simulink library "genset"  (R2014b)
settings: Solver=ode3  StartTime=0.0  StopTime=10.0  RelTol=1e-3
undefined symbols (not defined in the file): AFlowcontrol, AFn, generators, genset, i, Kappa1, ma0, magnitude, nr, pin0, swbId
libraries: goto x6, genset x3, simulink x2, switchboard x1
(part 2 of 2)

== system genset/GensetMV/Primover and generator/MVEM_TC/exhaustReceiver ==
  dm : Inport
  dE : Inport  Port=2
  dmb : Inport  Port=3
  dV : Inport  Port=4
  Bus Creator : BusCreator
  S-Function : S-Function  FunctionName=ThdynCVNV  Parameters=fs,m0,E0,mb0,V0  SFunctionModules=GetThdynCombGasZach.c GetPTF.c  EnableBusSupport=off
  pTFV : Outport
  wires:
  dE/1 -> S-Function/2
  dm/1 -> S-Function/1
  dmb/1 -> S-Function/3
  dV/1 -> S-Function/4
  S-Function/2 -> Bus Creator/2  "T"
  S-Function/1 -> Bus Creator/1  "p"
  S-Function/3 -> Bus Creator/3  "F"
  S-Function/4 -> Bus Creator/4  "V"
  Bus Creator/1 -> pTFV/1

== system genset/GensetMV/Primover and generator/MVEM_TC/pipe ==
  dm : Inport
  dE : Inport  Port=2
  dmb : Inport  Port=3
  dV : Inport  Port=4
  Bus Creator : BusCreator
  S-Function : S-Function  FunctionName=ThdynCVNV  Parameters=fs,m0,E0,mb0,V0  SFunctionModules=GetThdynCombGasZach.c GetPTF.c  EnableBusSupport=off
  pTFV : Outport
  wires:
  dE/1 -> S-Function/2
  dm/1 -> S-Function/1
  dmb/1 -> S-Function/3
  dV/1 -> S-Function/4
  S-Function/2 -> Bus Creator/2  "T"
  S-Function/1 -> Bus Creator/1  "p"
  S-Function/3 -> Bus Creator/3  "F"
  S-Function/4 -> Bus Creator/4  "V"
  Bus Creator/1 -> pTFV/1

== system genset/GensetMV/Primover and generator/Smoke Limiter MV/LP_T0_01 ==
  In1 : Inport
  Gain3 : Gain  Gain=100
  Integrator : Integrator  InitialCondition=T0AR
  Sum : Sum  Inputs=|+-
  Out1 : Outport
  wires:
  Integrator/1 -> Sum/2, Out1/1
  In1/1 -> Sum/1
  Sum/1 -> Gain3/1
  Gain3/1 -> Integrator/1

== system genset/GensetMV/Primover and generator/Smoke Limiter MV/LP_T0_1 ==
  In1 : Inport
  Gain3 : Gain  Gain=100
  Integrator : Integrator  InitialCondition=p0AR
  Sum : Sum  Inputs=|+-
  Out1 : Outport
  wires:
  Integrator/1 -> Sum/2, Out1/1
  In1/1 -> Sum/1
  Sum/1 -> Gain3/1
  Gain3/1 -> Integrator/1

== system genset/GensetMV/Primover and generator/Smoke Limiter MV/LP_T0_2 ==
  In1 : Inport
  Gain3 : Gain  Gain=100
  Integrator : Integrator  InitialCondition=p0AR/1e5*(p0AR/1e5*vol_eff_coeff(1) + vol_eff_coeff(2))+vol_eff_coeff(3)
  Sum : Sum  Inputs=|+-
  Out1 : Outport
  wires:
  Integrator/1 -> Sum/2, Out1/1
  In1/1 -> Sum/1
  Sum/1 -> Gain3/1
  Gain3/1 -> Integrator/1

== matlab function genset/GensetMV/Power calculation ==
  data: Z input; connected input; p output; E input; V input; q output; Vt output
function [p,q,Vt] = power(Z,connected,E,V)
%#codegen
if (connected)
Vt = V;
V = V/sqrt(3);
s = 3*V.*conj((E-V)./Z);
p = real(s);
q = imag(s);

else
p = 0;
q = 0;
Vt =E*sqrt(3);
end

== matlab function genset/GensetMV/Primover and generator/Electrical system ==
  data: umax input; p input size=1; q input; v input; genset_data input; te output; w input; pmax output size=1
function [te,pmax] = fcn(umax,p,q,v,genset_data,w)
r     = genset_data(1);
D     = genset_data(2);
p_max = genset_data(3);

te = (p+r*(p^2+q^2)/v^2)/w;
pmax = min((v/(1+r))*(-D*w^2+umax*w-r*q^2/v),p_max);

== matlab function genset/GensetMV/Primover and generator/Subsystem1/MATLAB Function ==
  data: u input; y output
function y = fcn(u)
%#codegen

y = anglemap(u);

== matlab function genset/GensetDC/MATLAB Function1 ==
  data: u input
function stopper(u)
%#codegen
if ( u < -1)
    error('Bus voltage calculations have been invalid for 1 second, stopping stimulation');
end

== matlab function genset/Genset/Power calculation ==
  data: Z input; connected input; p output; E input; V input; q output; Vt output
function [p,q,Vt] = power(Z,connected,E,V)
%#codegen
if (connected)
Vt = V;
V = V/sqrt(3);
s = 3*V.*conj((E-V)./Z);
p = real(s);
q = imag(s);

else
p = 0;
q = 0;
Vt =E*sqrt(3);
end

== matlab function genset/Genset/Primover and generator/Electrical system ==
  data: umax input; p input size=1; q input; v input; genset_data input; te output; w input; pmax output size=1
function [te,pmax] = fcn(umax,p,q,v,genset_data,w)
r     = genset_data(1);
D     = genset_data(2);
p_max = genset_data(3);

te = (p+r*(p^2+q^2)/v^2)/w;
pmax = min((v/(1+r))*(-D*w^2+umax*w-r*q^2/v),p_max);

== matlab function genset/Genset/Primover and generator/Subsystem1/MATLAB Function ==
  data: u input; y output
function y = fcn(u)
%#codegen

y = anglemap(u);

== matlab function genset/Genset/Primover and generator/turbo/MATLAB Function ==
  data: umax output; AFn parameter; ma0 parameter; AFlowcontrol parameter; u input; pin input; AF output; nr parameter
function [umax,AF] = AF(AFn,ma0,AFlowcontrol,u,pin,nr)
umax = (ma0(nr)+(1-ma0(nr))*pin)/AFlowcontrol(nr)*AFn(nr);
AF = (ma0(nr)+(1-ma0(nr))*pin)/u*AFn(nr);

== matlab function genset/Genset/Primover and generator/turbo/dead-band rate limiter/Delta ==
  data: p input; delta output
function delta = fcn(p)
%#codegen
if p<.33
    delta = .33-.303*p;
elseif p<.56
    delta = .3-.217*p;
elseif p<.74
    delta = -.068+.444*p;
else
    delta = .26;
end
